simulink library "PTOSim_Lib"  (Simulink 8.6)
settings: Solver=ode45  StartTime=0.0  StopTime=10.0  RelTol=1e-3
undefined symbols (not defined in the file or in its folder): pAeq, pAupper_limit, pBeq, pBupper_limit, ptosim, table
(part 1 of 2)
settings Model: RequirementInfo="{}  %GIDa_42666abb_d6d9_408c_ae24_f6520282b61c"  ForwardingTableString=||__slOldName__||Y:\MATLAB\PTO-Sim\Source\lib||__slNewName__||Y:\MATLAB\PTO-Sim\PassiveHydraulicPTO  Creator=sor  LastModifiedBy=yyu

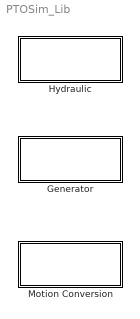
== system PTOSim_Lib ==
  " Generator" : Subsystem  RequirementInfo="{}  %GIDa_5439fdb4_7c29_433c_8677_23bf92e18f11"
  Hydraulic : Subsystem  RequirementInfo={} %GIDa_f12a42eb_b9cb_4818_b573_b7dee4183a3b
  Motion Conversion : Subsystem

== system PTOSim_Lib/ Generator ==
  Direct Drive Linear Generator : Subsystem  mask{ptosim=ptosim.pmLinearGenerator(1)}
      mask prompts: ptosim "Machine Name:"
      mask init:
      | if exist ('ptosim','var')
      |     h = [gcb '/To Workspace'];
      |     responseName = ['pmLinearGenerator' num2str(ptosim.number) '_out'];
      |     set_param(h,'VariableName',responseName);
      |     if ischar(ptosim.Rs)==1 ...
      |        || ischar(ptosim.Bfric)==1 ...
      |        || ischar(ptosim.tau_p)==1 ...
      |        || ischar(ptosim.lambda_fd)==1 ...
      |        || ischar(ptosim.Ls)==1 ...
      |        || ischar(ptosim.theta_d_0)==1 ...
      |        || ischar(ptosim.lambda_sq_0)==1 ...
      |        || ischar(ptosim.lambda_sd_0)==1 ...
      |        || ischar(ptosim.Rload) ==1
      |           error('One of the linear generator variables is undefined. For example, ptosim.pmLinearGenerator.variableName')
      |     end       
      | end
      | clear h responseName
  Direct Drive Rotary Generator : Subsystem  RequirementInfo="{}  %GIDa_f3580181_3e4e_42ef_9271_bab532422270"  mask{ptosim=ptosim.pmRotaryGenerator(1)}
      mask prompts: ptosim "Machine Name:"
      mask init:
      | if exist ('ptosim','var')
      |     h = [gcb '/To Workspace'];
      |     responseName = ['pmRotaryGenerator' num2str(ptosim.number) '_out'];
      |     set_param(h,'VariableName',responseName);
      |     if ischar(ptosim.Rs)==1 ...
      |        || ischar(ptosim.Bfric)==1 ...
      |        || ischar(ptosim.tau_p)==1 ...
      |        || ischar(ptosim.lambda_fd)==1 ...
      |        || ischar(ptosim.Ls)==1 ...
      |        || ischar(ptosim.theta_d_0)==1 ...
      |        || ischar(ptosim.lambda_sq_0)==1 ...
      |        || ischar(ptosim.lambda_sd_0)==1 ...
      |        || ischar(ptosim.Rload) ==1 ...
      |        || ischar(ptosim.radius) ==1
      |           error('One of the rotary generator variables is undefined. For example, ptosim.pmRotaryGenerator.variableName')
      |     end       
      | end
      | clear h responseName
  Rotary Generator Lookup Table : Subsystem  mask{ptosim=ptosim.rotaryGenerator(1)}
      mask prompts: ptosim "Generator Name"
      mask init:
      | if exist ('ptosim','var')
      |    h = [gcb '/To Workspace'];
      |    responseName = ['rotaryGenerator' num2str(ptosim.number) '_out'];
      |    set_param(h,'VariableName',responseName);
      |    if ischar(ptosim.TgenBase)==1 ...
      |       || ischar(ptosim.omegaBase)==1 ...
      |       || ischar(ptosim.driveEff)==1 ...
      |       || ischar(ptosim.desiredSpeed)==1
      |          error('One of the rotary generator variables is undefined. For example, ptosim.rotaryGenerator.variableName')
      |    end
      | end
      | clear h responseName

== system PTOSim_Lib/Hydraulic ==
  Accumulator : Subsystem  mask(PTO-Sim Element){ptosim=ptosim.accumulator(1)}
      mask prompts: ptosim "Accumulator Name:"
      mask init:
      | if exist('ptosim','var')
      |     h = [gcb '/To Workspace'];
      |     responseName = ['accumulator' num2str(ptosim.number) '_out'];
      |     set_param(h,'VariableName',responseName);
      |     if ischar(ptosim.VI0)==1 ...
      |             || ischar(ptosim.pIrated)==1 ...
      |             || ischar(ptosim.pIupper_limit)==1 ...
      |             || ischar(ptosim.pIlower_limit)==1 ...
      |             || ischar(ptosim.pIprecharge)==1 ...
      |             || ischar(ptosim.VImax)==1 ...
      |             || ischar(ptosim.VImin)==1 ...
      |             || ischar(ptosim.VIeq)==1 ...
      |             || ischar(ptosim.pIeq)==1 ...
      |             error('One of the accumulator variables is undefined. For example, ptosim.accumulator.variableName')
      |     end
      | end
      | clear h responseName
  Compressible Fluid Piston : Subsystem  mask{ptosim=ptosim.pistonCF(1)}
      mask prompts: ptosim "Piston Name:"
      mask init:
      | if exist ('ptosim','var')
      |     h = [gcb '/To Workspace'];
      |     responseName = ['pistonCF' num2str(ptosim.number) '_out'];
      |     set_param(h,'VariableName',responseName);
      |     
      |     if ischar(ptosim.Ap)==1 ...
      |       || ischar(ptosim.Vo)==1 ...
      |       || ischar(ptosim.Beta_e)==1 ...
      |       || ischar(ptosim.pAi)==1 ...
      |       || ischar(ptosim.pBi)==1 
      |          error('One of the piston variables is undefined. For example, ptosim.pistonCF.variableName')    
      |     end
      | end
      | clear h responseName
  "Hydraulic Motor " : Subsystem  mask{ptosim=ptosim.hydraulicMotor(1)}
      mask prompts: ptosim "Motor Name:"
      mask init:
      | if exist ('ptosim','var')
      |     h = [gcb '/To Workspace'];
      |     responseName = ['hydraulicMotor' num2str(ptosim.number) '_out'];
      |     set_param(h,'VariableName',responseName);
      |     if ischar(ptosim.angVelInit)==1 ...
      |        || ischar(ptosim.J)==1 ...
      |        || ischar(ptosim.fric)==1 ...
      |           error('One of the motor variables is undefined. For example, ptosim.hydraulicMotor.variableName')
      |     end       
      | end
      | clear h responseName
  Noncompressible Fluid Piston : Subsystem  mask{ptosim=ptosim.pistonNCF(1)}
      mask prompts: ptosim "Piston Name:"
      mask init:
      | if exist ('ptosim','var')
      |     h = [gcb '/To Workspace'];
      |     responseName = ['pistonNCF' num2str(ptosim.number) '_out'];
      |     set_param(h,'VariableName',responseName);
      |     if ischar(ptosim.topA)==1 ...
      |       || ischar(ptosim.botA)==1
      |          error('One of the piston variables is undefined. For example, ptosim.pistonNCF.variableName')
      |     end
      | end
      | clear h responseName
  Rectifying Check Valve : Subsystem  mask{ptosim=ptosim.checkValve(1)}
      mask prompts: ptosim "Valve Name:"
      mask init:
      | if exist ('ptosim','var')
      |     h = [gcb '/To Workspace'];
      |     responseName = ['checkValve' num2str(ptosim.number) '_out'];
      |     set_param(h,'VariableName',responseName);
      |     
      |     if ischar(ptosim.Cd)==1 ...
      |        || ischar(ptosim.Amax)==1 ...
      |        || ischar(ptosim.Amin)==1 ...
      |        || ischar(ptosim.pMax)==1 ...
      |        || ischar(ptosim.pMin)==1 ...
      |        || ischar(ptosim.rho)==1 ...
      |        || ischar(ptosim.k1)==1 ...
      |        || ischar(ptosim.k2)==1 
      |           error('One of valve variables is undefined. For exmaple, ptosim.checkValve.variableName')
      |     end
      | end
      | clear h responseName
  Rectifying Valve : Subsystem  mask{Parameter1=ptosim.valve(1)}
      mask init:
      | if exist ('ptosim','var')
      |     h = [gcb '/To Workspace'];
      |     responseName = ['valve' num2str(ptosim.number) '_out'];
      |     set_param(h,'VariableName',responseName);
      | end
      | clear h responseName

== system PTOSim_Lib/Motion Conversion ==
  Rotary to Linear Adjustable Rod : Subsystem  mask{ptosim=ptosim.motionMechanism(1)}
      mask prompts: ptosim "Telescope Name:"
      mask init:
      | if exist('ptosim','var')
      |     h = [gcb '/To Workspace'];
      |     responseName = ['motionMechanism' num2str(ptosim.number) '_out'];
      |     set_param(h,'VariableName',responseName);
      |     if ischar(ptosim.crank)==1 ...
      |             || ischar(ptosim.rodInit)==1 ...
      |             || ischar(ptosim.offset)==1 ...
      |             error('One of the rotary to linear adjustable rod variables is undefined. For example, ptosim.motionMechanism.variableName')
      |     end
      | end
      | clear h responseName
  Rotary to Linear Crank : Subsystem  mask{ptosim=ptosim.motionMechanism(1)}
      mask prompts: ptosim "Crank Name:"
      mask init:
      | if exist('ptosim','var')
      |     h = [gcb '/To Workspace'];
      |     responseName = ['motionMechanism' num2str(ptosim.number) '_out'];
      |     set_param(h,'VariableName',responseName);
      |     if ischar(ptosim.crank)==1 ...
      |             || ischar(ptosim.rodLength)==1 ...
      |             || ischar(ptosim.offset)==1 ...
      |             error('One of the rotary to linear crank variables is undefined. For example, ptosim.motionMechanism.variableName')
      |     end
      | end
      | clear h responseName

== system PTOSim_Lib/ Generator/Direct Drive Linear Generator ==
  note: In this model d-axis aligned with rotor magnets
      | in other words lambda_fq = 0
  note: Ls = 3/2*Lsinglephase
  vel : Inport
  ABC2DQ1 : Subsystem
  ABC2DQ2 : Subsystem
  Bus Creator : BusCreator  Inputs=11
  Demux : Demux  Outputs=3
  Demux1 : Demux  Outputs=3
  Gain4 : Gain  Gain=-1
  Gain5 : Gain  Gain=2*pi/(2*ptosim.tau_p)
  Integrator2 : Integrator  InitialCondition=ptosim.theta_d_0
  Load : Subsystem
  Losses : Subsystem
  Product1 : Product
  Subsystem : Subsystem
  Sum : Sum
  Terminator3 : Terminator
  To Workspace : ToWorkspace  VariableName=pmLinearGenerator1_out  SaveFormat=Structure With Time  SampleTime=-1
      settings: Decimation=round(simu.dtOut/simu.dt,0)
  force : Outport
  wires:
  ABC2DQ2/1(DQ) -> Subsystem/1(vsdq)  "vsdq"
  ABC2DQ1/1(abc) -> Demux/1, Load/1(Iabc)  "Iabc"
  Gain5/1 -> Subsystem/2(wd), Integrator2/1  "wsyn"
  Integrator2/1 -> ABC2DQ2/1(theta_d), ABC2DQ1/1(theta_d)
  Product1/1 -> Gain4/1
  Gain4/1 -> Bus Creator/1, Terminator3/1  "absPower"
  Subsystem/1(Fem) -> Sum/2
  Subsystem/2(isdq) -> ABC2DQ1/2(dq)
  Losses/1(friceForce) -> Bus Creator/3, Sum/1  "fricForce"
  Sum/1 -> Bus Creator/2, Product1/2, force/1  "force"
  Load/1(Vabc) -> Demux1/1, ABC2DQ2/2(ABC)  "Vabc"
  vel/1 -> Bus Creator/10, Losses/1(vel), Product1/1, Gain5/1  "vel"
  Bus Creator/1 -> To Workspace/1
  Demux/1 -> Bus Creator/4  "Ia"
  Demux/2 -> Bus Creator/5  "Ib"
  Demux/3 -> Bus Creator/6  "Ic"
  Demux1/1 -> Bus Creator/7  "Va"
  Demux1/2 -> Bus Creator/8  "Vb"
  Demux1/3 -> Bus Creator/9  "Vc"
  Load/2(elecPower) -> Bus Creator/11  "elecPower"

== system PTOSim_Lib/ Generator/Direct Drive Rotary Generator ==
  note: In this model d-axis aligned with rotor magnets
      | in other words lambda_fq = 0
  note: Ls = 3/2*Lsinglephase
  vel : Inport
  ABC2DQ1 : Subsystem
  ABC2DQ2 : Subsystem
  Bus Creator : BusCreator  Inputs=11
  Demux : Demux  Outputs=3
  Demux1 : Demux  Outputs=3
  Gain4 : Gain  Gain=-1
  Gain5 : Gain  Gain=2*pi*ptosim.radius/(2*ptosim.tau_p)
  Integrator2 : Integrator  InitialCondition=ptosim.theta_d_0
  Load : Subsystem
  Losses : Subsystem
  Product1 : Product
  Subsystem : Subsystem
  Sum : Sum
  Terminator3 : Terminator
  To Workspace : ToWorkspace  VariableName=pmRotaryGenerator1_out  SaveFormat=Structure With Time  SampleTime=-1
      settings: Decimation=round(simu.dtOut/simu.dt,0)
  torque : Outport
  wires:
  ABC2DQ2/1(DQ) -> Subsystem/1(vsdq)  "vsdq"
  ABC2DQ1/1(abc) -> Demux/1, Load/1(Iabc)  "Iabc"
  Gain5/1 -> Integrator2/1, Subsystem/2(wd)  "wsyn"
  Integrator2/1 -> ABC2DQ2/1(theta_d), ABC2DQ1/1(theta_d)
  Product1/1 -> Gain4/1
  Gain4/1 -> Bus Creator/1, Terminator3/1  "absPower"
  Subsystem/1(Tem) -> Sum/2
  Subsystem/2(isdq) -> ABC2DQ1/2(dq)
  Losses/1(fricTorque) -> Bus Creator/3, Sum/1  "fricTorque"
  Sum/1 -> Bus Creator/2, Product1/2, torque/1  "torque"
  Load/1(Vabc) -> Demux1/1, ABC2DQ2/2(ABC)  "Vabc"
  vel/1 -> Losses/1(vel), Product1/1, Gain5/1, Bus Creator/10  "vel"
  Bus Creator/1 -> To Workspace/1
  Demux/1 -> Bus Creator/4  "Ia"
  Demux/2 -> Bus Creator/5  "Ib"
  Demux/3 -> Bus Creator/6  "Ic"
  Demux1/1 -> Bus Creator/7  "Va"
  Demux1/2 -> Bus Creator/8  "Vb"
  Demux1/3 -> Bus Creator/9  "Vc"
  Load/2(elecPower) -> Bus Creator/11  "elecPower"

== system PTOSim_Lib/ Generator/Rotary Generator Lookup Table ==
  delPress : Inport
  motorVol : Inport  Port=2
  angVel : Inport  Port=3
  Base Motor Torque : Gain  Gain=-1/ptosim.TgenBase
  Base Motor Torque1 : Gain  Gain=1/ptosim.omegaBase
  Base Motor Torque2 : Gain  Gain=ptosim.driveEff
  Base Motor Torque3 : Gain  Gain=1/100
  Base Motor Torque4 : Gain  Gain=1.05
  Bus Creator : BusCreator  Inputs=2
  Constant47 : Constant  Value=ptosim.desiredSpeed
  Divide1 : Product  Inputs=*/
  PM p.u. Efficiency Lookup Table : Lookup_n-D  BreakpointsForDimension1=table.Tpu(:,1)  BreakpointsForDimension2=table.omegapu(1,:)  Table=table.eff  InterpMethod=Flat  InputSameDT=on
  Product{,1..3} (4 alike) : Product  RndMeth=Zero
  To Workspace : ToWorkspace  VariableName=rotaryGenerator1_out  SaveFormat=Structure With Time  SampleTime=-1
      settings: Decimation=round(simu.dtOut/simu.dt,0)
  genTorque : Outport
  wires:
  angVel/1 -> Product2/2, Product/2, Base Motor Torque1/1
  Product2/1 -> Product/1, Base Motor Torque/1, genTorque/1
  Bus Creator/1 -> To Workspace/1
  Base Motor Torque/1 -> PM p.u. Efficiency Lookup Table/1  "torquePU"
  Base Motor Torque1/1 -> PM p.u. Efficiency Lookup Table/2  "omegaPU"
  PM p.u. Efficiency Lookup Table/1 -> Base Motor Torque3/1
  Base Motor Torque3/1 -> Product1/2  "genEff"
  Product/1 -> Product1/1, Bus Creator/2  "genPower"
  Product1/1 -> Base Motor Torque2/1
  Base Motor Torque2/1 -> Bus Creator/1  "elecPower"
  Divide1/1 -> Product2/1
  delPress/1 -> Product3/1
  motorVol/1 -> Product3/2
  Product3/1 -> Divide1/1
  Constant47/1 -> Base Motor Torque4/1
  Base Motor Torque4/1 -> Divide1/2

== system PTOSim_Lib/Hydraulic/Accumulator ==
  volFlowM : Inport
  volFlowAccum : Inport  Port=2
  Bus Creator : BusCreator  Inputs=2
  Constant : Constant
  Constant3 : Constant  Value=ptosim.pIprecharge
  Constant4 : Constant  Value=ptosim.VI0
  Divide : Product  Inputs=*/
  Divide1 : Product  Inputs=*/
  Exponent : Constant  Value=1.4
  Integrator4 : Integrator  InitialCondition=ptosim.VIeq
  Math Function : Math  Operator=pow  SaturateOnIntegerOverflow=on
  Sum : Sum  Inputs=-+
  Sum2 : Sum
  To Workspace : ToWorkspace  VariableName=accum_out  SaveFormat=Structure With Time  SampleTime=-1
      settings: Decimation=round(simu.dtOut/simu.dt,0)
  pressure : Outport
  wires:
  Sum2/1 -> Integrator4/1
  Integrator4/1 -> Bus Creator/2, Divide/1  "volume"
  Constant4/1 -> Divide/2
  Constant/1 -> Sum/2
  Divide/1 -> Sum/1
  Exponent/1 -> Math Function/2
  Sum/1 -> Math Function/1
  Math Function/1 -> Divide1/2
  Constant3/1 -> Divide1/1
  Divide1/1 -> pressure/1, Bus Creator/1  "pressure"
  volFlowAccum/1 -> Sum2/2
  volFlowM/1 -> Sum2/1
  Bus Creator/1 -> To Workspace/1

== system PTOSim_Lib/Hydraulic/Compressible Fluid Piston ==
  pos : Inport
  vel : Inport  Port=2
  volFlowTop : Inport  Port=3
  volFlowBottom : Inport  Port=4
  Bus Creator : BusCreator  Inputs=4
  Gain1 : Gain  Gain=-1
  Gain6 : Gain  Gain=ptosim.Ap
  Gain7 : Gain  Gain=ptosim.Ap
  Pressure Bottom : Subsystem
  Pressure Top : Subsystem
  Product : Product
  Sum4 : Sum  Inputs=-+
  To Workspace : ToWorkspace  VariableName=pistonCF1_out  SaveFormat=Structure With Time  SampleTime=-1
      settings: Decimation=round(simu.dtOut/simu.dt,0)
  force : Outport
  topPressure : Outport  Port=2
  bottomPressure : Outport  Port=3
  wires:
  Pressure Top/1(topPressure) -> Sum4/1, topPressure/1
  Pressure Bottom/1(bottomPressure) -> bottomPressure/1, Sum4/2
  Gain7/1 -> Pressure Bottom/3(volFLowP), Pressure Top/3(volFlowP)
  pos/1 -> Bus Creator/3, Pressure Bottom/1(pos), Pressure Top/1(pos)  "pos"
  vel/1 -> Bus Creator/4, Product/2, Gain7/1  "vel"
  Sum4/1 -> Gain6/1
  Gain6/1 -> Bus Creator/2, force/1, Product/1  "force"
  volFlowBottom/1 -> Pressure Bottom/2(volFlowBottom)
  volFlowTop/1 -> Pressure Top/2(volFlowTop)
  Bus Creator/1 -> To Workspace/1
  Gain1/1 -> Bus Creator/1  "absPower"
  Product/1 -> Gain1/1

== system PTOSim_Lib/Hydraulic/Hydraulic Motor  ==
  highPressure : Inport
  lowPressure : Inport  Port=2
  genTorque : Inport  Port=3
  Bus Creator : BusCreator  Inputs=2
  Constant47 : Constant  Value=ptosim.J
  Divide1 : Product  Inputs=*/
  Gain1 : Gain  Gain=ptosim.fric
  Gain4 : Gain  Gain=-1
  Integrator1 : Integrator  InitialCondition=ptosim.angVelInit
  Interpreted MATLAB Function : MATLABFcn  MATLABFcn=variableMotorVolume
  Product : Product
  Product1 : Product
  Sum1 : Sum  Inputs=+--
  Sum2 : Sum  Inputs=+-
  To Workspace : ToWorkspace  VariableName=hydraulicMotor1_out  SaveFormat=Structure With Time  SampleTime=-1
      settings: Decimation=round(simu.dtOut/simu.dt,0)
  delPress : Outport
  motorVol : Outport  Port=2
  angVel : Outport  Port=3
  volFlowMHigh : Outport  Port=4
  volFlowMLow : Outport  Port=5
  wires:
  Interpreted MATLAB Function/1 -> motorVol/1, Product/2, Product1/2
  Sum2/1 -> delPress/1, Product/1, Interpreted MATLAB Function/1
  Gain1/1 -> Sum1/3
  genTorque/1 -> Sum1/2, Gain1/1
  Bus Creator/1 -> To Workspace/1
  Gain4/1 -> volFlowMHigh/1
  lowPressure/1 -> Sum2/2
  highPressure/1 -> Sum2/1
  Integrator1/1 -> angVel/1, Product1/1, Bus Creator/1  "angVel"
  Divide1/1 -> Integrator1/1
  Constant47/1 -> Divide1/2
  Sum1/1 -> Divide1/1
  Product/1 -> Sum1/1
  Product1/1 -> volFlowMLow/1, Gain4/1, Bus Creator/2  "volFlowM"

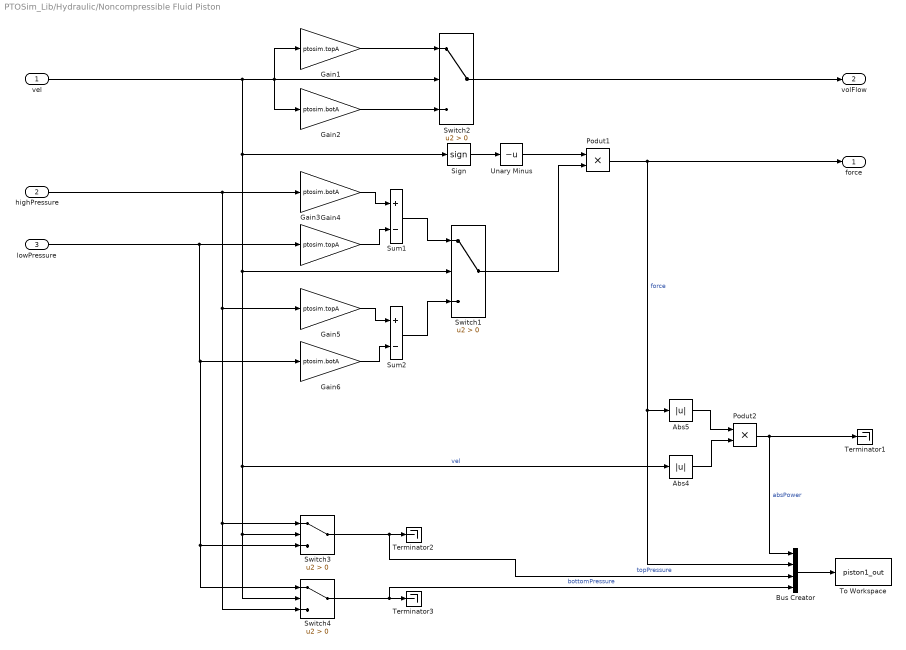
== system PTOSim_Lib/Hydraulic/Noncompressible Fluid Piston ==
  vel : Inport
  highPressure : Inport  Port=2
  lowPressure : Inport  Port=3
  Abs4 : Abs
  Abs5 : Abs
  Bus Creator : BusCreator  Inputs=4
  Gain1 : Gain  Gain=ptosim.topA
  Gain2 : Gain  Gain=ptosim.botA
  Gain3 : Gain  Gain=ptosim.topA
  Gain4 : Gain  Gain=ptosim.botA
  Gain5 : Gain  Gain=ptosim.topA
  Gain6 : Gain  Gain=ptosim.botA
  Podut1 : Product  RndMeth=Zero
  Podut2 : Product  RndMeth=Zero
  Sign : Signum
  Sum1 : Sum  Inputs=+-
  Sum2 : Sum  Inputs=+-
  Switch{1..4} (4 alike) : Switch  Criteria=u2 > Threshold
  Terminator1 : Terminator
  Terminator2 : Terminator
  Terminator3 : Terminator
  To Workspace : ToWorkspace  VariableName=piston1_out  SaveFormat=Structure With Time  SampleTime=-1
      settings: Decimation=round(simu.dtOut/simu.dt,0)
  Unary Minus : UnaryMinus
  force : Outport
  volFlow : Outport  Port=2
  wires:
  vel/1 -> Switch1/2, Switch4/2, Switch3/2, Abs4/1, Sign/1, Gain2/1, Switch2/2, Gain1/1  "vel"
  Podut2/1 -> Bus Creator/1, Terminator1/1  "absPower"
  Abs5/1 -> Podut2/1
  Abs4/1 -> Podut2/2
  Gain1/1 -> Switch2/1
  Gain2/1 -> Switch2/3
  Sum1/1 -> Switch1/1
  Podut1/1 -> force/1, Bus Creator/2, Abs5/1  "force"
  Gain4/1 -> Sum1/1
  Gain3/1 -> Sum1/2
  highPressure/1 -> Gain5/1, Switch3/1, Switch4/3, Gain4/1
  lowPressure/1 -> Switch4/1, Switch3/3, Gain6/1, Gain3/1
  Gain5/1 -> Sum2/1
  Gain6/1 -> Sum2/2
  Sum2/1 -> Switch1/3
  Sign/1 -> Unary Minus/1
  Unary Minus/1 -> Podut1/1
  Switch1/1 -> Podut1/2
  Switch3/1 -> Bus Creator/3, Terminator2/1  "topPressure"
  Switch4/1 -> Bus Creator/4, Terminator3/1  "bottomPressure"
  Switch2/1 -> volFlow/1
  Bus Creator/1 -> To Workspace/1

== system PTOSim_Lib/Hydraulic/Rectifying Check Valve ==
  topPressure : Inport
  bottomPressure : Inport  Port=2
  highPressure : Inport  Port=3
  lowPressure : Inport  Port=4
  Bus Creator : BusCreator  Inputs=4
  Subsystem : Subsystem
  Subsystem1 : Subsystem
  Subsystem2 : Subsystem
  Subsystem3 : Subsystem
  Sum1 : Sum  Inputs=-+
  Sum2 : Sum
  Sum3 : Sum  Inputs=--
  Sum4 : Sum  Inputs=-+
  To Workspace : ToWorkspace  VariableName=valve1_out  SaveFormat=Structure With Time  SampleTime=-1
      settings: Decimation=round(simu.dtOut/simu.dt,0)
  volFlowTop : Outport
  volFlowBottom : Outport  Port=2
  volFlowHigh : Outport  Port=3
  volFlowLow : Outport  Port=4
  wires:
  topPressure/1 -> Subsystem3/2(topPressure), Subsystem/1(topPressure)
  bottomPressure/1 -> Subsystem2/2(bottomPressure), Subsystem1/1(bottomPressure)
  highPressure/1 -> Subsystem1/2(highPressure), Subsystem/2(highPressure)
  lowPressure/1 -> Subsystem2/1(lowPressure), Subsystem3/1(lowPressure)
  Subsystem3/1(volFlow4) -> Bus Creator/4, Sum4/2, Sum3/2  "volFlow4"
  Subsystem2/1(volFlow3) -> Bus Creator/3, Sum3/1, Sum1/2  "volFlow3"
  Subsystem1/1(volFlow2) -> Bus Creator/2, Sum2/2, Sum1/1  "volFlow2"
  Subsystem/1(volFlow1) -> Bus Creator/1, Sum2/1, Sum4/1  "volFlow1"
  Sum4/1 -> volFlowTop/1
  Sum1/1 -> volFlowBottom/1
  Sum2/1 -> volFlowHigh/1
  Sum3/1 -> volFlowLow/1
  Bus Creator/1 -> To Workspace/1

== system PTOSim_Lib/Hydraulic/Rectifying Valve ==
  volFlow : Inport
  Abs1 : Abs
  To Workspace : ToWorkspace  VariableName=valve1_out  SaveFormat=Structure With Time  SampleTime=-1
      settings: Decimation=round(simu.dtOut/simu.dt,0)
  electric generator control1 : Gain  Gain=-1
  volFlowHigh : Outport
  volFlowLow : Outport  Port=2
  wires:
  Abs1/1 -> To Workspace/1, volFlowHigh/1, electric generator control1/1  "volFlow"
  electric generator control1/1 -> volFlowLow/1
  volFlow/1 -> Abs1/1

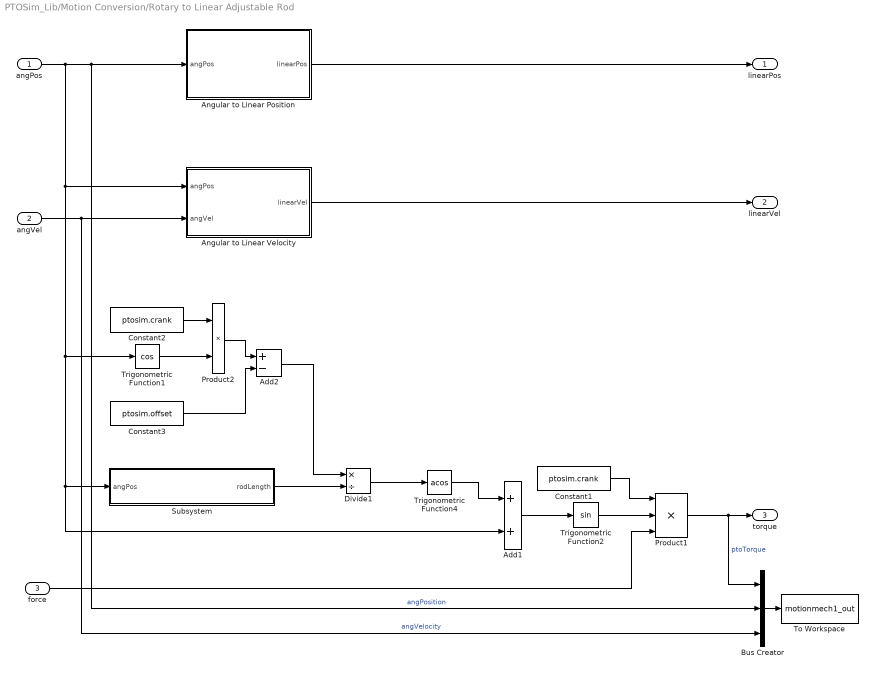
== system PTOSim_Lib/Motion Conversion/Rotary to Linear Adjustable Rod ==
  angPos : Inport
  angVel : Inport  Port=2
  force : Inport  Port=3
  Add1 : Sum
  Add2 : Sum  Inputs=+-
  Angular to Linear Position : Subsystem
  Angular to Linear Velocity : Subsystem
  Bus Creator : BusCreator  Inputs=3
  Constant1 : Constant  Value=ptosim.crank
  Constant2 : Constant  Value=ptosim.crank
  Constant3 : Constant  Value=ptosim.offset
  Divide1 : Product  Inputs=*/
  Product1 : Product  Inputs=***
  Product2 : Product  Inputs=**
  Subsystem : Subsystem
  To Workspace : ToWorkspace  VariableName=motionmech1_out  SaveFormat=Structure With Time  SampleTime=-1
      settings: Decimation=round(simu.dtOut/simu.dt,0)
  Trigonometric Function1 : Trigonometry  Operator=cos
  Trigonometric Function2 : Trigonometry
  Trigonometric Function4 : Trigonometry  Operator=acos
  linearPos : Outport
  linearVel : Outport  Port=2
  torque : Outport  Port=3
  wires:
  Angular to Linear Position/1(linearPos) -> linearPos/1
  angVel/1 -> Bus Creator/3, Angular to Linear Velocity/2(angVel)  "angVelocity"
  Angular to Linear Velocity/1(linearVel) -> linearVel/1
  Subsystem/1(rodLength) -> Divide1/2
  Divide1/1 -> Trigonometric Function4/1
  Trigonometric Function4/1 -> Add1/1
  Add1/1 -> Trigonometric Function2/1
  Constant1/1 -> Product1/1
  Trigonometric Function2/1 -> Product1/2
  force/1 -> Product1/3
  Product1/1 -> Bus Creator/1, torque/1  "ptoTorque"
  angPos/1 -> Angular to Linear Velocity/1(angPos), Trigonometric Function1/1, Subsystem/1(angPos), Add1/2, Bus Creator/2, Angular to Linear Position/1(angPos)  "angPosition"
  Add2/1 -> Divide1/1
  Constant2/1 -> Product2/1
  Trigonometric Function1/1 -> Product2/2
  Product2/1 -> Add2/1
  Constant3/1 -> Add2/2
  Bus Creator/1 -> To Workspace/1

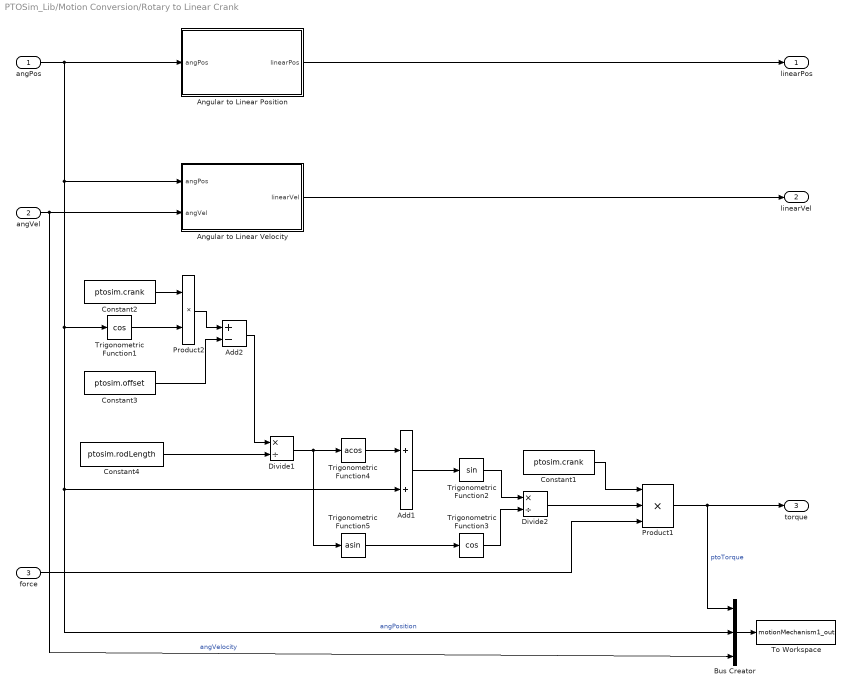
== system PTOSim_Lib/Motion Conversion/Rotary to Linear Crank ==
  angPos : Inport
  angVel : Inport  Port=2
  force : Inport  Port=3
  Add1 : Sum
  Add2 : Sum  Inputs=+-
  Angular to Linear Position : Subsystem
  Angular to Linear Velocity : Subsystem
  Bus Creator : BusCreator  Inputs=3
  Constant1 : Constant  Value=ptosim.crank
  Constant2 : Constant  Value=ptosim.crank
  Constant3 : Constant  Value=ptosim.offset
  Constant4 : Constant  Value=ptosim.rodLength
  Divide1 : Product  Inputs=*/
  Divide2 : Product  Inputs=*/
  Product1 : Product  Inputs=***
  Product2 : Product  Inputs=**
  To Workspace : ToWorkspace  VariableName=motionMechanism1_out  SaveFormat=Structure With Time  SampleTime=-1
      settings: Decimation=round(simu.dtOut/simu.dt,0)
  Trigonometric Function1 : Trigonometry  Operator=cos
  Trigonometric Function2 : Trigonometry
  Trigonometric Function3 : Trigonometry  Operator=cos
  Trigonometric Function4 : Trigonometry  Operator=acos
  Trigonometric Function5 : Trigonometry  Operator=asin
  linearPos : Outport
  linearVel : Outport  Port=2
  torque : Outport  Port=3
  wires:
  Angular to Linear Position/1(linearPos) -> linearPos/1
  angVel/1 -> Bus Creator/3, Angular to Linear Velocity/2(angVel)  "angVelocity"
  Angular to Linear Velocity/1(linearVel) -> linearVel/1
  Constant4/1 -> Divide1/2
  Divide1/1 -> Trigonometric Function5/1, Trigonometric Function4/1
  Trigonometric Function4/1 -> Add1/1
  Add1/1 -> Trigonometric Function2/1
  Constant1/1 -> Product1/1
  Product1/1 -> Bus Creator/1, torque/1  "ptoTorque"
  angPos/1 -> Angular to Linear Velocity/1(angPos), Trigonometric Function1/1, Bus Creator/2, Add1/2, Angular to Linear Position/1(angPos)  "angPosition"
  Add2/1 -> Divide1/1
  Constant2/1 -> Product2/1
  Trigonometric Function1/1 -> Product2/2
  Product2/1 -> Add2/1
  Constant3/1 -> Add2/2
  Trigonometric Function2/1 -> Divide2/1
  Trigonometric Function3/1 -> Divide2/2
  Trigonometric Function5/1 -> Trigonometric Function3/1
  Divide2/1 -> Product1/2
  force/1 -> Product1/3
  Bus Creator/1 -> To Workspace/1

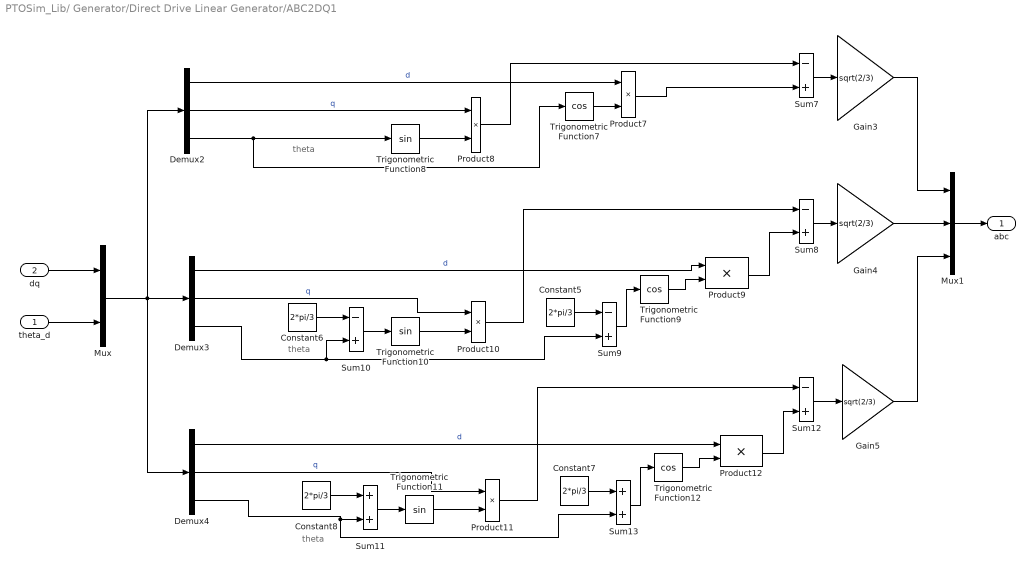
== system PTOSim_Lib/ Generator/Direct Drive Linear Generator/ABC2DQ1 ==
  note: theta
  note: theta
  note: theta
  theta_d : Inport
  dq : Inport  Port=2
  Constant{5..8} (4 alike) : Constant  Value=2*pi/3
  Demux2 : Demux  Outputs=3
  Demux3 : Demux  Outputs=3
  Demux4 : Demux  Outputs=3
  Gain3 : Gain  Gain=sqrt(2/3)  SaturateOnIntegerOverflow=on  OutDataTypeStr=Inherit: Same as input  ParamDataTypeStr=Inherit: Same as input
  Gain4 : Gain  Gain=sqrt(2/3)  SaturateOnIntegerOverflow=on  OutDataTypeStr=Inherit: Same as input  ParamDataTypeStr=Inherit: Same as input
  Gain5 : Gain  Gain=sqrt(2/3)  SaturateOnIntegerOverflow=on  OutDataTypeStr=Inherit: Same as input  ParamDataTypeStr=Inherit: Same as input
  Mux : Mux  Inputs=2
  Mux1 : Mux  Inputs=3
  Product{7..12} (6 alike) : Product  SaturateOnIntegerOverflow=on  InputSameDT=on  OutDataTypeStr=Inherit: Same as first input
  Sum{7..10,12} (5 alike) : Sum  Inputs=-+  SaturateOnIntegerOverflow=on  InputSameDT=on  OutDataTypeStr=Inherit: Same as first input
  Sum11 : Sum  SaturateOnIntegerOverflow=on  InputSameDT=on  OutDataTypeStr=Inherit: Same as first input
  Sum13 : Sum  SaturateOnIntegerOverflow=on  InputSameDT=on  OutDataTypeStr=Inherit: Same as first input
  Trigonometric Function10 : Trigonometry
  Trigonometric Function11 : Trigonometry
  Trigonometric Function12 : Trigonometry  Operator=cos
  Trigonometric Function7 : Trigonometry  Operator=cos
  Trigonometric Function8 : Trigonometry
  Trigonometric Function9 : Trigonometry  Operator=cos
  abc : Outport
  wires:
  Mux1/1 -> abc/1
  dq/1 -> Mux/1
  theta_d/1 -> Mux/2
  Mux/1 -> Demux4/1, Demux2/1, Demux3/1
  Trigonometric Function7/1 -> Product7/2
  Demux2/1 -> Product7/1  "d"
  Product7/1 -> Sum7/2
  Product8/1 -> Sum7/1
  Demux2/3 -> Trigonometric Function8/1, Trigonometric Function7/1
  Demux2/2 -> Product8/1  "q"
  Trigonometric Function9/1 -> Product9/2
  Demux3/1 -> Product9/1  "d"
  Product9/1 -> Sum8/2
  Product10/1 -> Sum8/1
  Demux3/3 -> Sum10/2, Sum9/2
  Trigonometric Function10/1 -> Product10/2
  Demux3/2 -> Product10/1  "q"
  Sum9/1 -> Trigonometric Function9/1
  Constant5/1 -> Sum9/1
  Sum10/1 -> Trigonometric Function10/1
  Constant6/1 -> Sum10/1
  Trigonometric Function12/1 -> Product12/2
  Demux4/1 -> Product12/1  "d"
  Product12/1 -> Sum12/2
  Product11/1 -> Sum12/1
  Demux4/3 -> Sum13/2, Sum11/2
  Trigonometric Function11/1 -> Product11/2
  Demux4/2 -> Product11/1  "q"
  Sum13/1 -> Trigonometric Function12/1
  Constant7/1 -> Sum13/1
  Sum11/1 -> Trigonometric Function11/1
  Constant8/1 -> Sum11/1
  Sum7/1 -> Gain3/1
  Sum8/1 -> Gain4/1
  Sum12/1 -> Gain5/1
  Gain3/1 -> Mux1/1
  Gain4/1 -> Mux1/2
  Gain5/1 -> Mux1/3
  Trigonometric Function8/1 -> Product8/2

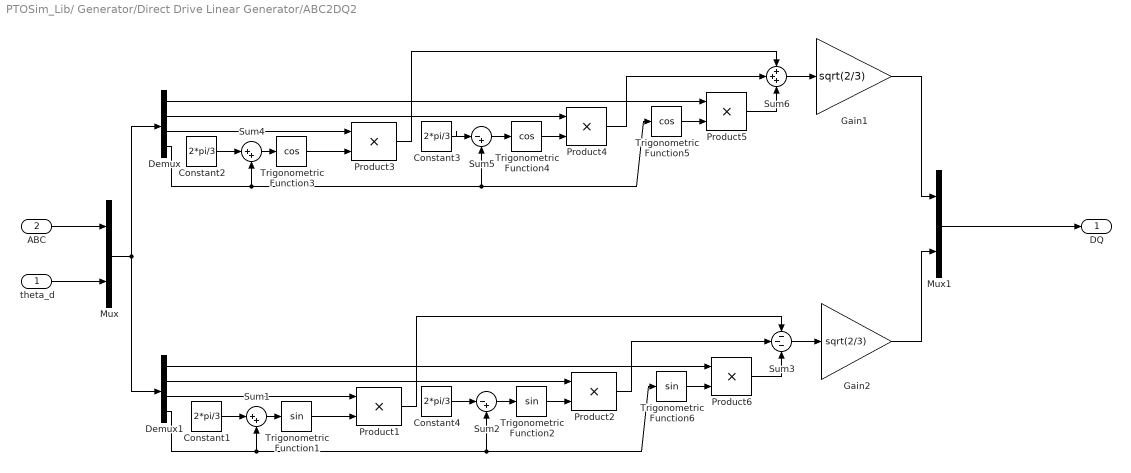
== system PTOSim_Lib/ Generator/Direct Drive Linear Generator/ABC2DQ2 ==
  theta_d : Inport
  ABC : Inport  Port=2
  Constant{1..4} (4 alike) : Constant  Value=2*pi/3
  Demux : Demux
  Demux1 : Demux
  Gain1 : Gain  Gain=sqrt(2/3)  SaturateOnIntegerOverflow=on  OutDataTypeStr=Inherit: Same as input  ParamDataTypeStr=Inherit: Same as input
  Gain2 : Gain  Gain=sqrt(2/3)  SaturateOnIntegerOverflow=on  OutDataTypeStr=Inherit: Same as input  ParamDataTypeStr=Inherit: Same as input
  Mux : Mux  Inputs=2
  Mux1 : Mux  Inputs=2
  Product{1..6} (6 alike) : Product  SaturateOnIntegerOverflow=on  InputSameDT=on  OutDataTypeStr=Inherit: Same as first input
  Sum1 : Sum  Inputs=|++  SaturateOnIntegerOverflow=on  InputSameDT=on  OutDataTypeStr=Inherit: Same as first input
  Sum2 : Sum  Inputs=|-+  SaturateOnIntegerOverflow=on  InputSameDT=on  OutDataTypeStr=Inherit: Same as first input
  Sum3 : Sum  Inputs=---  SaturateOnIntegerOverflow=on  InputSameDT=on  OutDataTypeStr=Inherit: Same as first input
  Sum4 : Sum  Inputs=|++  SaturateOnIntegerOverflow=on  InputSameDT=on  OutDataTypeStr=Inherit: Same as first input
  Sum5 : Sum  Inputs=|-+  SaturateOnIntegerOverflow=on  InputSameDT=on  OutDataTypeStr=Inherit: Same as first input
  Sum6 : Sum  Inputs=+++  SaturateOnIntegerOverflow=on  InputSameDT=on  OutDataTypeStr=Inherit: Same as first input
  Trigonometric Function1 : Trigonometry
  Trigonometric Function2 : Trigonometry
  Trigonometric Function3 : Trigonometry  Operator=cos
  Trigonometric Function4 : Trigonometry  Operator=cos
  Trigonometric Function5 : Trigonometry  Operator=cos
  Trigonometric Function6 : Trigonometry
  DQ : Outport
  wires:
  Mux1/1 -> DQ/1
  Product5/1 -> Sum6/3
  Constant2/1 -> Sum4/1
  Sum5/1 -> Trigonometric Function4/1
  Trigonometric Function4/1 -> Product4/2
  Trigonometric Function5/1 -> Product5/2
  Constant3/1 -> Sum5/1
  Sum6/1 -> Gain1/1
  Product3/1 -> Sum6/1
  Product4/1 -> Sum6/2
  Trigonometric Function3/1 -> Product3/2
  Gain1/1 -> Mux1/1
  ABC/1 -> Mux/1
  theta_d/1 -> Mux/2
  Demux/1 -> Product5/1
  Demux/2 -> Product4/1
  Demux/3 -> Product3/1
  Demux/4 -> Sum5/2, Trigonometric Function5/1, Sum4/2
  Mux/1 -> Demux/1, Demux1/1
  Sum4/1 -> Trigonometric Function3/1
  Product6/1 -> Sum3/3
  Constant1/1 -> Sum1/1
  Sum2/1 -> Trigonometric Function2/1
  Trigonometric Function2/1 -> Product2/2
  Trigonometric Function6/1 -> Product6/2
  Constant4/1 -> Sum2/1
  Sum3/1 -> Gain2/1
  Product1/1 -> Sum3/1
  Product2/1 -> Sum3/2
  Trigonometric Function1/1 -> Product1/2
  Gain2/1 -> Mux1/2
  Demux1/1 -> Product6/1
  Demux1/2 -> Product2/1
  Demux1/3 -> Product1/1
  Demux1/4 -> Sum1/2, Trigonometric Function6/1, Sum2/2
  Sum1/1 -> Trigonometric Function1/1

== system PTOSim_Lib/ Generator/Direct Drive Linear Generator/Load ==
  Iabc : Inport
  Gain : Gain  Gain=-1
  Gain1 : Gain  Gain=ptosim.Rload
  Product : Product
  Sum of Elements : Sum  Inputs=+
  Vabc : Outport
  elecPower : Outport  Port=2
  wires:
  Gain/1 -> elecPower/1  "elecPower"
  Gain1/1 -> Product/1, Vabc/1
  Product/1 -> Sum of Elements/1
  Iabc/1 -> Gain1/1, Product/2
  Sum of Elements/1 -> Gain/1

== system PTOSim_Lib/ Generator/Direct Drive Linear Generator/Losses ==
  vel : Inport
  Gain : Gain  Gain=ptosim.Bfric
  friceForce : Outport
  wires:
  vel/1 -> Gain/1
  Gain/1 -> friceForce/1

== system PTOSim_Lib/ Generator/Direct Drive Linear Generator/Subsystem ==
  vsdq : Inport
  wd : Inport  Port=2
  Add : Sum  Inputs=+-+
  Add1 : Sum  Inputs=--+
  Demux2 : Demux  Outputs=2
  Fcn : Fcn  Expr=( u(1) - ptosim.lambda_fd ) / ptosim.Ls
  Gain : Gain  Gain=1/ptosim.Ls
  Gain1 : Gain  Gain=pi/ptosim.tau_p*ptosim.lambda_fd
  Gain2 : Gain  Gain=ptosim.Rs
  Gain3 : Gain  Gain=ptosim.Rs
  Integrator : Integrator  InitialCondition=ptosim.lambda_sd_0
  Integrator1 : Integrator  InitialCondition=ptosim.lambda_sq_0
  Mux : Mux  Inputs=2
  Product : Product  RndMeth=Zero
  Product1 : Product  RndMeth=Zero
  Fem : Outport
  isdq : Outport  Port=2
  wires:
  Add/1 -> Integrator/1  "d_dt_lambda_sd"
  Integrator/1 -> Product1/2, Fcn/1  "lambda_sd"
  Fcn/1 -> Gain3/1, Mux/1  "isd"
  Product/1 -> Add/1
  Add1/1 -> Integrator1/1  "d_dt_lambda_sq"
  Integrator1/1 -> Gain/1, Product/2  "lambda_sq"
  wd/1 -> Product1/1, Product/1
  Gain/1 -> Gain2/1, Mux/2, Gain1/1  "isq"
  Product1/1 -> Add1/1
  Demux2/1 -> Add/3  "vsd"
  Demux2/2 -> Add1/3  "vsq"
  vsdq/1 -> Demux2/1  "vsdq"
  Gain3/1 -> Add/2  "isd_Rs"
  Gain2/1 -> Add1/2
  Mux/1 -> isdq/1  "isdq"
  Gain1/1 -> Fem/1

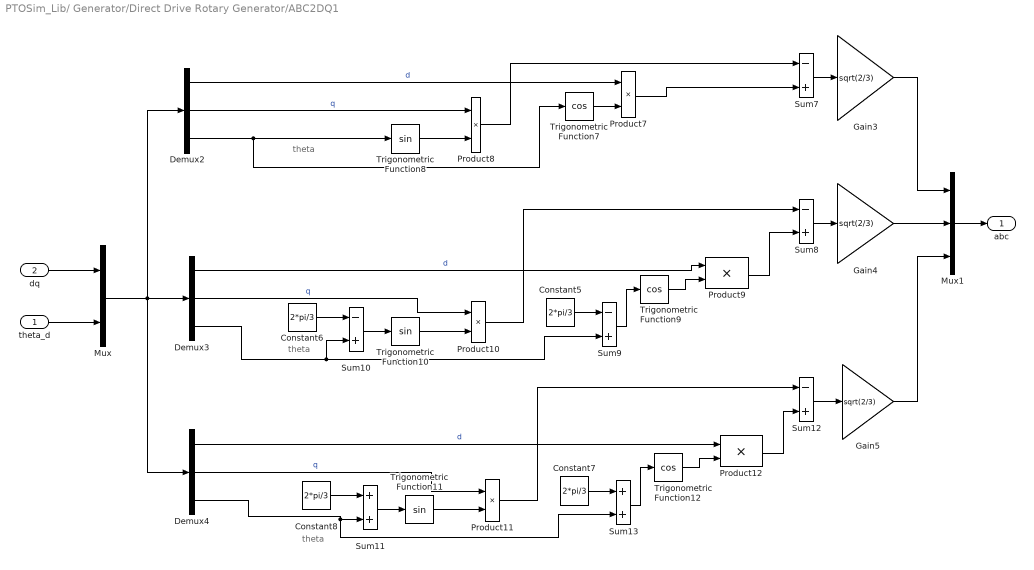
== system PTOSim_Lib/ Generator/Direct Drive Rotary Generator/ABC2DQ1 ==
  note: theta
  note: theta
  note: theta
  theta_d : Inport
  dq : Inport  Port=2
  Constant{5..8} (4 alike) : Constant  Value=2*pi/3
  Demux2 : Demux  Outputs=3
  Demux3 : Demux  Outputs=3
  Demux4 : Demux  Outputs=3
  Gain3 : Gain  Gain=sqrt(2/3)  SaturateOnIntegerOverflow=on  OutDataTypeStr=Inherit: Same as input  ParamDataTypeStr=Inherit: Same as input
  Gain4 : Gain  Gain=sqrt(2/3)  SaturateOnIntegerOverflow=on  OutDataTypeStr=Inherit: Same as input  ParamDataTypeStr=Inherit: Same as input
  Gain5 : Gain  Gain=sqrt(2/3)  SaturateOnIntegerOverflow=on  OutDataTypeStr=Inherit: Same as input  ParamDataTypeStr=Inherit: Same as input
  Mux : Mux  Inputs=2
  Mux1 : Mux  Inputs=3
  Product{7..12} (6 alike) : Product  SaturateOnIntegerOverflow=on  InputSameDT=on  OutDataTypeStr=Inherit: Same as first input
  Sum{7..10,12} (5 alike) : Sum  Inputs=-+  SaturateOnIntegerOverflow=on  InputSameDT=on  OutDataTypeStr=Inherit: Same as first input
  Sum11 : Sum  SaturateOnIntegerOverflow=on  InputSameDT=on  OutDataTypeStr=Inherit: Same as first input
  Sum13 : Sum  SaturateOnIntegerOverflow=on  InputSameDT=on  OutDataTypeStr=Inherit: Same as first input
  Trigonometric Function10 : Trigonometry
  Trigonometric Function11 : Trigonometry
  Trigonometric Function12 : Trigonometry  Operator=cos
  Trigonometric Function7 : Trigonometry  Operator=cos
  Trigonometric Function8 : Trigonometry
  Trigonometric Function9 : Trigonometry  Operator=cos
  abc : Outport
  wires:
  Mux1/1 -> abc/1
  dq/1 -> Mux/1
  theta_d/1 -> Mux/2
  Mux/1 -> Demux4/1, Demux2/1, Demux3/1
  Trigonometric Function7/1 -> Product7/2
  Demux2/1 -> Product7/1  "d"
  Product7/1 -> Sum7/2
  Product8/1 -> Sum7/1
  Demux2/3 -> Trigonometric Function8/1, Trigonometric Function7/1
  Demux2/2 -> Product8/1  "q"
  Trigonometric Function9/1 -> Product9/2
  Demux3/1 -> Product9/1  "d"
  Product9/1 -> Sum8/2
  Product10/1 -> Sum8/1
  Demux3/3 -> Sum10/2, Sum9/2
  Trigonometric Function10/1 -> Product10/2
  Demux3/2 -> Product10/1  "q"
  Sum9/1 -> Trigonometric Function9/1
  Constant5/1 -> Sum9/1
  Sum10/1 -> Trigonometric Function10/1
  Constant6/1 -> Sum10/1
  Trigonometric Function12/1 -> Product12/2
  Demux4/1 -> Product12/1  "d"
  Product12/1 -> Sum12/2
  Product11/1 -> Sum12/1
  Demux4/3 -> Sum13/2, Sum11/2
  Trigonometric Function11/1 -> Product11/2
  Demux4/2 -> Product11/1  "q"
  Sum13/1 -> Trigonometric Function12/1
  Constant7/1 -> Sum13/1
  Sum11/1 -> Trigonometric Function11/1
  Constant8/1 -> Sum11/1
  Sum7/1 -> Gain3/1
  Sum8/1 -> Gain4/1
  Sum12/1 -> Gain5/1
  Gain3/1 -> Mux1/1
  Gain4/1 -> Mux1/2
  Gain5/1 -> Mux1/3
  Trigonometric Function8/1 -> Product8/2

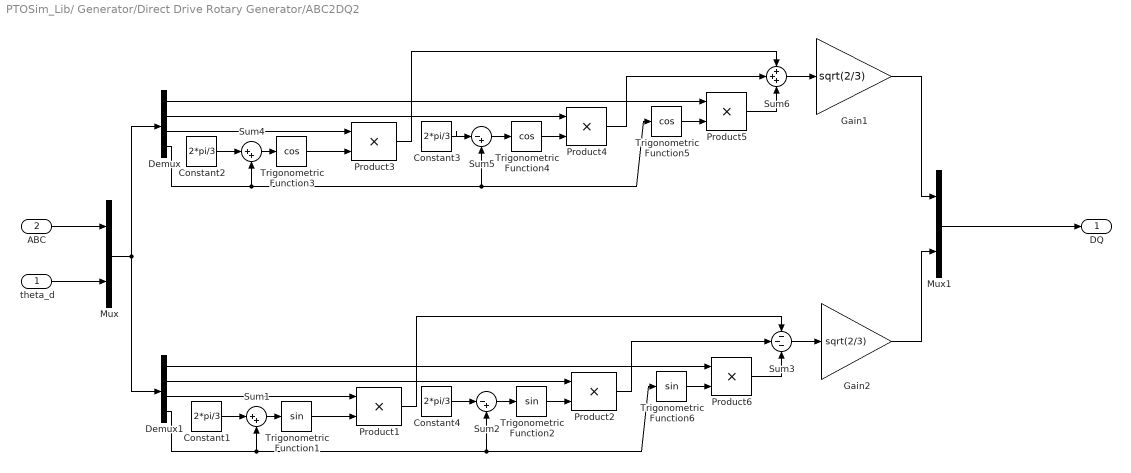
== system PTOSim_Lib/ Generator/Direct Drive Rotary Generator/ABC2DQ2 ==
  theta_d : Inport
  ABC : Inport  Port=2
  Constant{1..4} (4 alike) : Constant  Value=2*pi/3
  Demux : Demux
  Demux1 : Demux
  Gain1 : Gain  Gain=sqrt(2/3)  SaturateOnIntegerOverflow=on  OutDataTypeStr=Inherit: Same as input  ParamDataTypeStr=Inherit: Same as input
  Gain2 : Gain  Gain=sqrt(2/3)  SaturateOnIntegerOverflow=on  OutDataTypeStr=Inherit: Same as input  ParamDataTypeStr=Inherit: Same as input
  Mux : Mux  Inputs=2
  Mux1 : Mux  Inputs=2
  Product{1..6} (6 alike) : Product  SaturateOnIntegerOverflow=on  InputSameDT=on  OutDataTypeStr=Inherit: Same as first input
  Sum1 : Sum  Inputs=|++  SaturateOnIntegerOverflow=on  InputSameDT=on  OutDataTypeStr=Inherit: Same as first input
  Sum2 : Sum  Inputs=|-+  SaturateOnIntegerOverflow=on  InputSameDT=on  OutDataTypeStr=Inherit: Same as first input
  Sum3 : Sum  Inputs=---  SaturateOnIntegerOverflow=on  InputSameDT=on  OutDataTypeStr=Inherit: Same as first input
  Sum4 : Sum  Inputs=|++  SaturateOnIntegerOverflow=on  InputSameDT=on  OutDataTypeStr=Inherit: Same as first input
  Sum5 : Sum  Inputs=|-+  SaturateOnIntegerOverflow=on  InputSameDT=on  OutDataTypeStr=Inherit: Same as first input
  Sum6 : Sum  Inputs=+++  SaturateOnIntegerOverflow=on  InputSameDT=on  OutDataTypeStr=Inherit: Same as first input
  Trigonometric Function1 : Trigonometry
  Trigonometric Function2 : Trigonometry
  Trigonometric Function3 : Trigonometry  Operator=cos
  Trigonometric Function4 : Trigonometry  Operator=cos
  Trigonometric Function5 : Trigonometry  Operator=cos
  Trigonometric Function6 : Trigonometry
  DQ : Outport
  wires:
  Mux1/1 -> DQ/1
  Product5/1 -> Sum6/3
  Constant2/1 -> Sum4/1
  Sum5/1 -> Trigonometric Function4/1
  Trigonometric Function4/1 -> Product4/2
  Trigonometric Function5/1 -> Product5/2
  Constant3/1 -> Sum5/1
  Sum6/1 -> Gain1/1
  Product3/1 -> Sum6/1
  Product4/1 -> Sum6/2
  Trigonometric Function3/1 -> Product3/2
  Gain1/1 -> Mux1/1
  ABC/1 -> Mux/1
  theta_d/1 -> Mux/2
  Demux/1 -> Product5/1
  Demux/2 -> Product4/1
  Demux/3 -> Product3/1
  Demux/4 -> Sum5/2, Trigonometric Function5/1, Sum4/2
  Mux/1 -> Demux/1, Demux1/1
  Sum4/1 -> Trigonometric Function3/1
  Product6/1 -> Sum3/3
  Constant1/1 -> Sum1/1
  Sum2/1 -> Trigonometric Function2/1
  Trigonometric Function2/1 -> Product2/2
  Trigonometric Function6/1 -> Product6/2
  Constant4/1 -> Sum2/1
  Sum3/1 -> Gain2/1
  Product1/1 -> Sum3/1
  Product2/1 -> Sum3/2
  Trigonometric Function1/1 -> Product1/2
  Gain2/1 -> Mux1/2
  Demux1/1 -> Product6/1
  Demux1/2 -> Product2/1
  Demux1/3 -> Product1/1
  Demux1/4 -> Sum1/2, Trigonometric Function6/1, Sum2/2
  Sum1/1 -> Trigonometric Function1/1

== system PTOSim_Lib/ Generator/Direct Drive Rotary Generator/Load ==
  Iabc : Inport
  Gain : Gain  Gain=-1
  Gain1 : Gain  Gain=ptosim.Rload
  Product : Product
  Sum of Elements : Sum  Inputs=+
  Vabc : Outport
  elecPower : Outport  Port=2
  wires:
  Gain/1 -> elecPower/1  "elecPower"
  Gain1/1 -> Product/1, Vabc/1
  Product/1 -> Sum of Elements/1
  Iabc/1 -> Gain1/1, Product/2
  Sum of Elements/1 -> Gain/1

== system PTOSim_Lib/ Generator/Direct Drive Rotary Generator/Losses ==
  vel : Inport
  Gain : Gain  Gain=ptosim.Bfric
  fricTorque : Outport
  wires:
  vel/1 -> Gain/1
  Gain/1 -> fricTorque/1

== system PTOSim_Lib/ Generator/Direct Drive Rotary Generator/Subsystem ==
  vsdq : Inport
  wd : Inport  Port=2
  Add : Sum  Inputs=+-+
  Add1 : Sum  Inputs=--+
  Demux2 : Demux  Outputs=2
  Fcn : Fcn  Expr=( u(1) - ptosim.lambda_fd ) / ptosim.Ls
  Gain : Gain  Gain=1/ptosim.Ls
  Gain1 : Gain  Gain=(pi*ptosim.radius/ptosim.tau_p)*ptosim.lambda_fd
  Gain2 : Gain  Gain=ptosim.Rs
  Gain3 : Gain  Gain=ptosim.Rs
  Integrator : Integrator  InitialCondition=ptosim.lambda_sd_0
  Integrator1 : Integrator  InitialCondition=ptosim.lambda_sq_0
  Mux : Mux  Inputs=2
  Product : Product  RndMeth=Zero
  Product1 : Product  RndMeth=Zero
  Tem : Outport
  isdq : Outport  Port=2
  wires:
  Add/1 -> Integrator/1  "d_dt_lambda_sd"
  Integrator/1 -> Product1/2, Fcn/1  "lambda_sd"
  Fcn/1 -> Gain3/1, Mux/1  "isd"
  Product/1 -> Add/1
  Add1/1 -> Integrator1/1  "d_dt_lambda_sq"
  Integrator1/1 -> Gain/1, Product/2  "lambda_sq"
  wd/1 -> Product1/1, Product/1
  Gain/1 -> Gain2/1, Mux/2, Gain1/1  "isq"
  Product1/1 -> Add1/1
  Demux2/1 -> Add/3  "vsd"
  Demux2/2 -> Add1/3  "vsq"
  vsdq/1 -> Demux2/1  "vsdq"
  Gain3/1 -> Add/2  "isd_Rs"
  Gain2/1 -> Add1/2
  Mux/1 -> isdq/1  "isdq"
  Gain1/1 -> Tem/1

== system PTOSim_Lib/Hydraulic/Compressible Fluid Piston/Pressure Bottom ==
  pos : Inport
  volFlowBottom : Inport  Port=2
  volFLowP : Inport  Port=3
  Constant1 : Constant  Value=ptosim.Vo
  Divide1 : Product  Inputs=*/
  Gain4 : Gain  Gain=ptosim.Beta_e
  Gain5 : Gain  Gain=ptosim.Ap
  Integrator3 : Integrator  InitialCondition=ptosim.pBi  UpperSaturationLimit=pBupper_limit  LowerSaturationLimit=pBeq
  Sum2 : Sum  Inputs=+-
  Sum3 : Sum
  bottomPressure : Outport
  wires:
  volFLowP/1 -> Sum2/2
  Integrator3/1 -> bottomPressure/1
  volFlowBottom/1 -> Sum2/1
  Divide1/1 -> Integrator3/1
  Sum3/1 -> Divide1/2
  Gain4/1 -> Divide1/1
  Constant1/1 -> Sum3/2
  Gain5/1 -> Sum3/1
  pos/1 -> Gain5/1
  Sum2/1 -> Gain4/1

== system PTOSim_Lib/Hydraulic/Compressible Fluid Piston/Pressure Top ==
  pos : Inport
  volFlowTop : Inport  Port=2
  volFlowP : Inport  Port=3
  Constant : Constant  Value=ptosim.Vo
  Divide : Product  Inputs=*/
  Gain1 : Gain  Gain=ptosim.Beta_e
  Gain2 : Gain  Gain=ptosim.Ap
  Integrator2 : Integrator  InitialCondition=ptosim.pAi  UpperSaturationLimit=pAupper_limit  LowerSaturationLimit=pAeq
  Sum : Sum
  Sum1 : Sum  Inputs=-+
  topPressure : Outport
  wires:
  volFlowP/1 -> Sum/2
  Integrator2/1 -> topPressure/1
  Divide/1 -> Integrator2/1
  volFlowTop/1 -> Sum/1
  Sum1/1 -> Divide/2
  Gain1/1 -> Divide/1
  Constant/1 -> Sum1/2
  Gain2/1 -> Sum1/1
  pos/1 -> Gain2/1
  Sum/1 -> Gain1/1

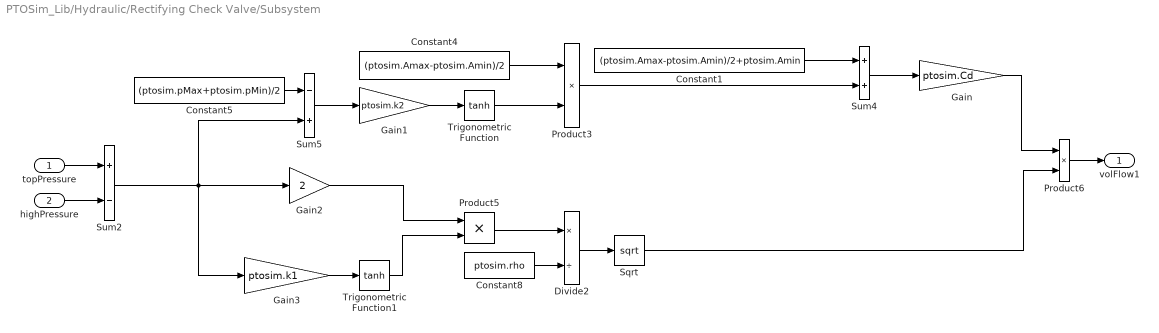
== system PTOSim_Lib/Hydraulic/Rectifying Check Valve/Subsystem ==
  topPressure : Inport
  highPressure : Inport  Port=2
  Constant1 : Constant  Value=(ptosim.Amax-ptosim.Amin)/2+ptosim.Amin
  Constant4 : Constant  Value=(ptosim.Amax-ptosim.Amin)/2
  Constant5 : Constant  Value=(ptosim.pMax+ptosim.pMin)/2
  Constant8 : Constant  Value=ptosim.rho
  Divide2 : Product  Inputs=*/
  Gain : Gain  Gain=ptosim.Cd
  Gain1 : Gain  Gain=ptosim.k2
  Gain2 : Gain  Gain=2
  Gain3 : Gain  Gain=ptosim.k1
  Product3 : Product
  Product5 : Product
  Product6 : Product
  Sqrt : Sqrt  SaturateOnIntegerOverflow=on
  Sum2 : Sum  Inputs=+-
  Sum4 : Sum
  Sum5 : Sum  Inputs=-+
  Trigonometric Function : Trigonometry  Operator=tanh
  Trigonometric Function1 : Trigonometry  Operator=tanh
  volFlow1 : Outport
  wires:
  Gain1/1 -> Trigonometric Function/1
  Trigonometric Function/1 -> Product3/2
  Product3/1 -> Sum4/2
  Sum5/1 -> Gain1/1
  Sum4/1 -> Gain/1
  Gain3/1 -> Trigonometric Function1/1
  Gain2/1 -> Product5/1
  Trigonometric Function1/1 -> Product5/2
  Sqrt/1 -> Product6/2
  Gain/1 -> Product6/1
  Constant8/1 -> Divide2/2
  Product5/1 -> Divide2/1
  Divide2/1 -> Sqrt/1
  topPressure/1 -> Sum2/1
  highPressure/1 -> Sum2/2
  Product6/1 -> volFlow1/1
  Constant4/1 -> Product3/1
  Constant5/1 -> Sum5/1
  Constant1/1 -> Sum4/1
  Sum2/1 -> Gain3/1, Sum5/2, Gain2/1

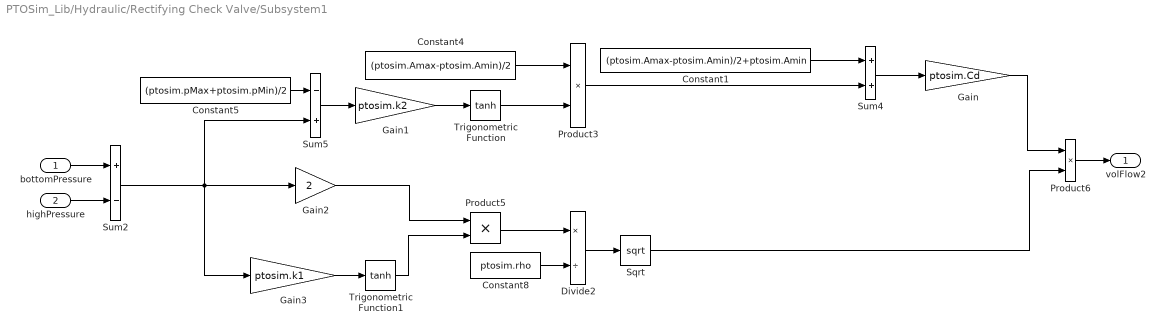
== system PTOSim_Lib/Hydraulic/Rectifying Check Valve/Subsystem1 ==
  bottomPressure : Inport
  highPressure : Inport  Port=2
  Constant1 : Constant  Value=(ptosim.Amax-ptosim.Amin)/2+ptosim.Amin
  Constant4 : Constant  Value=(ptosim.Amax-ptosim.Amin)/2
  Constant5 : Constant  Value=(ptosim.pMax+ptosim.pMin)/2
  Constant8 : Constant  Value=ptosim.rho
  Divide2 : Product  Inputs=*/
  Gain : Gain  Gain=ptosim.Cd
  Gain1 : Gain  Gain=ptosim.k2
  Gain2 : Gain  Gain=2
  Gain3 : Gain  Gain=ptosim.k1
  Product3 : Product
  Product5 : Product
  Product6 : Product
  Sqrt : Sqrt  SaturateOnIntegerOverflow=on
  Sum2 : Sum  Inputs=+-
  Sum4 : Sum
  Sum5 : Sum  Inputs=-+
  Trigonometric Function : Trigonometry  Operator=tanh
  Trigonometric Function1 : Trigonometry  Operator=tanh
  volFlow2 : Outport
  wires:
  Gain1/1 -> Trigonometric Function/1
  Trigonometric Function/1 -> Product3/2
  Product3/1 -> Sum4/2
  Sum5/1 -> Gain1/1
  Sum4/1 -> Gain/1
  Gain3/1 -> Trigonometric Function1/1
  Gain2/1 -> Product5/1
  Trigonometric Function1/1 -> Product5/2
  Sqrt/1 -> Product6/2
  Gain/1 -> Product6/1
  Constant8/1 -> Divide2/2
  Product5/1 -> Divide2/1
  Divide2/1 -> Sqrt/1
  bottomPressure/1 -> Sum2/1
  highPressure/1 -> Sum2/2
  Product6/1 -> volFlow2/1
  Constant4/1 -> Product3/1
  Constant5/1 -> Sum5/1
  Constant1/1 -> Sum4/1
  Sum2/1 -> Gain3/1, Sum5/2, Gain2/1

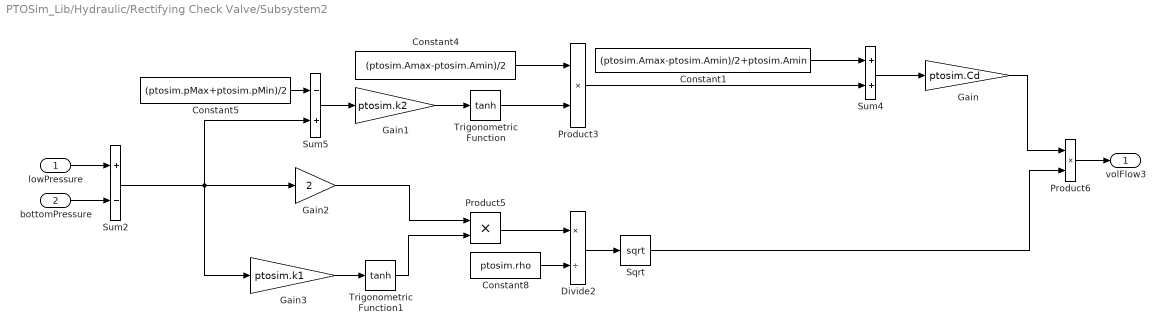
== system PTOSim_Lib/Hydraulic/Rectifying Check Valve/Subsystem2 ==
  lowPressure : Inport
  bottomPressure : Inport  Port=2
  Constant1 : Constant  Value=(ptosim.Amax-ptosim.Amin)/2+ptosim.Amin
  Constant4 : Constant  Value=(ptosim.Amax-ptosim.Amin)/2
  Constant5 : Constant  Value=(ptosim.pMax+ptosim.pMin)/2
  Constant8 : Constant  Value=ptosim.rho
  Divide2 : Product  Inputs=*/
  Gain : Gain  Gain=ptosim.Cd
  Gain1 : Gain  Gain=ptosim.k2
  Gain2 : Gain  Gain=2
  Gain3 : Gain  Gain=ptosim.k1
  Product3 : Product
  Product5 : Product
  Product6 : Product
  Sqrt : Sqrt  SaturateOnIntegerOverflow=on
  Sum2 : Sum  Inputs=+-
  Sum4 : Sum
  Sum5 : Sum  Inputs=-+
  Trigonometric Function : Trigonometry  Operator=tanh
  Trigonometric Function1 : Trigonometry  Operator=tanh
  volFlow3 : Outport
  wires:
  Gain1/1 -> Trigonometric Function/1
  Trigonometric Function/1 -> Product3/2
  Product3/1 -> Sum4/2
  Sum5/1 -> Gain1/1
  Sum4/1 -> Gain/1
  Gain3/1 -> Trigonometric Function1/1
  Gain2/1 -> Product5/1
  Trigonometric Function1/1 -> Product5/2
  Sqrt/1 -> Product6/2
  Gain/1 -> Product6/1
  Constant8/1 -> Divide2/2
  Product5/1 -> Divide2/1
  Divide2/1 -> Sqrt/1
  lowPressure/1 -> Sum2/1
  bottomPressure/1 -> Sum2/2
  Product6/1 -> volFlow3/1
  Constant4/1 -> Product3/1
  Constant5/1 -> Sum5/1
  Constant1/1 -> Sum4/1
  Sum2/1 -> Gain3/1, Sum5/2, Gain2/1

== system PTOSim_Lib/Hydraulic/Rectifying Check Valve/Subsystem3 ==
  lowPressure : Inport
  topPressure : Inport  Port=2
  Constant1 : Constant  Value=(ptosim.Amax-ptosim.Amin)/2+ptosim.Amin
  Constant4 : Constant  Value=(ptosim.Amax-ptosim.Amin)/2
  Constant5 : Constant  Value=(ptosim.pMax+ptosim.pMin)/2
  Constant8 : Constant  Value=ptosim.rho
  Divide2 : Product  Inputs=*/
  Gain : Gain  Gain=ptosim.Cd
  Gain1 : Gain  Gain=ptosim.k2
  Gain2 : Gain  Gain=2
  Gain3 : Gain  Gain=ptosim.k1
  Product3 : Product
  Product5 : Product
  Product6 : Product
  Sqrt : Sqrt  SaturateOnIntegerOverflow=on
  Sum2 : Sum  Inputs=+-
  Sum4 : Sum
  Sum5 : Sum  Inputs=-+
  Trigonometric Function : Trigonometry  Operator=tanh
  Trigonometric Function1 : Trigonometry  Operator=tanh
  volFlow4 : Outport
  wires:
  Gain1/1 -> Trigonometric Function/1
  Trigonometric Function/1 -> Product3/2
  Product3/1 -> Sum4/2
  Sum5/1 -> Gain1/1
  Sum4/1 -> Gain/1
  Gain3/1 -> Trigonometric Function1/1
  Gain2/1 -> Product5/1
  Trigonometric Function1/1 -> Product5/2
  Sqrt/1 -> Product6/2
  Gain/1 -> Product6/1
  Constant8/1 -> Divide2/2
  Product5/1 -> Divide2/1
  Divide2/1 -> Sqrt/1
  lowPressure/1 -> Sum2/1
  topPressure/1 -> Sum2/2
  Product6/1 -> volFlow4/1
  Constant4/1 -> Product3/1
  Constant5/1 -> Sum5/1
  Constant1/1 -> Sum4/1
  Sum2/1 -> Gain3/1, Sum5/2, Gain2/1

== system PTOSim_Lib/Motion Conversion/Rotary to Linear Adjustable Rod/Angular to Linear Position ==
  angPos : Inport
  Add1 : Sum  Inputs=+-
  Add2 : Sum  Inputs=+-
  Add5 : Sum
  Add6 : Sum  Inputs=+-
  Constant1 : Constant  Value=ptosim.rodInit
  Constant2 : Constant  Value=ptosim.crank
  Constant3 : Constant  Value=ptosim.offset
  Constant7 : Constant  Value=ptosim.crank
  Distance btw flap joint & rod joint along x-axis : Subsystem
  Math Function1 : Math  Operator=square  SaturateOnIntegerOverflow=on
  Math Function6 : Math  Operator=square  SaturateOnIntegerOverflow=on
  Product1 : Product  Inputs=**
  Product7 : Product  Inputs=**
  Sqrt2 : Sqrt  SaturateOnIntegerOverflow=on
  Trigonometric Function1 : Trigonometry  Operator=cos
  Trigonometric Function5 : Trigonometry
  linearPos : Outport
  wires:
  angPos/1 -> Trigonometric Function5/1, Trigonometric Function1/1
  Add1/1 -> linearPos/1
  Add2/1 -> Math Function1/1
  Trigonometric Function5/1 -> Product7/2
  Product7/1 -> Add6/2
  Add6/1 -> Math Function6/1
  Math Function6/1 -> Add5/2
  Add5/1 -> Sqrt2/1
  Sqrt2/1 -> Add1/2
  Constant1/1 -> Add1/1
  Constant2/1 -> Product1/1
  Trigonometric Function1/1 -> Product1/2
  Product1/1 -> Add2/1
  Constant3/1 -> Add2/2
  Math Function1/1 -> Add5/1
  Constant7/1 -> Product7/1
  Distance btw flap joint & rod joint along x-axis/1(d) -> Add6/1

== system PTOSim_Lib/Motion Conversion/Rotary to Linear Adjustable Rod/Angular to Linear Velocity ==
  angPos : Inport
  angVel : Inport  Port=2
  Add1 : Sum  Inputs=+-
  Add2 : Sum  Inputs=+-
  Add3 : Sum
  Constant1 : Constant  Value=ptosim.crank
  Constant2 : Constant  Value=ptosim.crank
  Constant3 : Constant  Value=ptosim.offset
  Constant7 : Constant  Value=ptosim.crank
  Distance btw flap joint & rod joint along x-axis : Subsystem
  Divide1 : Product  Inputs=*/
  Product1 : Product  Inputs=**
  Product2 : Product  Inputs=***
  Product3 : Product  Inputs=**
  Product4 : Product  Inputs=***
  Product7 : Product  Inputs=**
  Subsystem : Subsystem
  Trigonometric Function1 : Trigonometry  Operator=cos
  Trigonometric Function2 : Trigonometry  Operator=cos
  Trigonometric Function5 : Trigonometry
  linearVel : Outport
  wires:
  Add2/1 -> Product2/1
  Constant2/1 -> Product1/1
  Trigonometric Function1/1 -> Product1/2
  Product1/1 -> Add2/1
  Constant3/1 -> Add2/2
  Trigonometric Function5/1 -> Product7/2
  Product7/1 -> Add1/1, Product2/2
  Constant7/1 -> Product7/1
  angVel/1 -> Product2/3, Product4/1
  Distance btw flap joint & rod joint along x-axis/1(d) -> Add1/2
  Constant1/1 -> Product3/1
  Trigonometric Function2/1 -> Product3/2
  Product3/1 -> Product4/3
  angPos/1 -> Trigonometric Function5/1, Trigonometric Function2/1, Trigonometric Function1/1, Subsystem/1(angPos)
  Add1/1 -> Product4/2
  Subsystem/1(rodLength) -> Divide1/2
  Product2/1 -> Add3/1
  Product4/1 -> Add3/2
  Add3/1 -> Divide1/1
  Divide1/1 -> linearVel/1
